simulink model "EX4zadanie2"  (R2023b)
settings: Solver=FixedStepDiscrete  StartTime=0.0  StopTime=0.0  RelTol=1e-3
libraries: CPOiS_SourcesSinks x10, CPOiS_Filters x6, CPOiS_DataManipulation_DataTypeConversion x6, CPOiS_DataManipulation_IntroduceNoise x2
settings Model: Creator=kkarkosz  LastModifiedBy=alyskawa

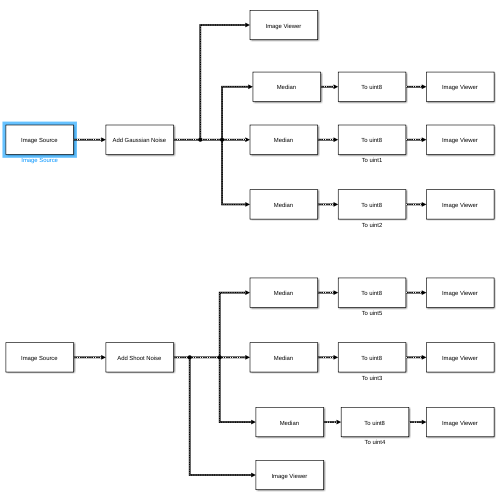
[thumbnail: Simulink's stored preview of the top-level diagram]
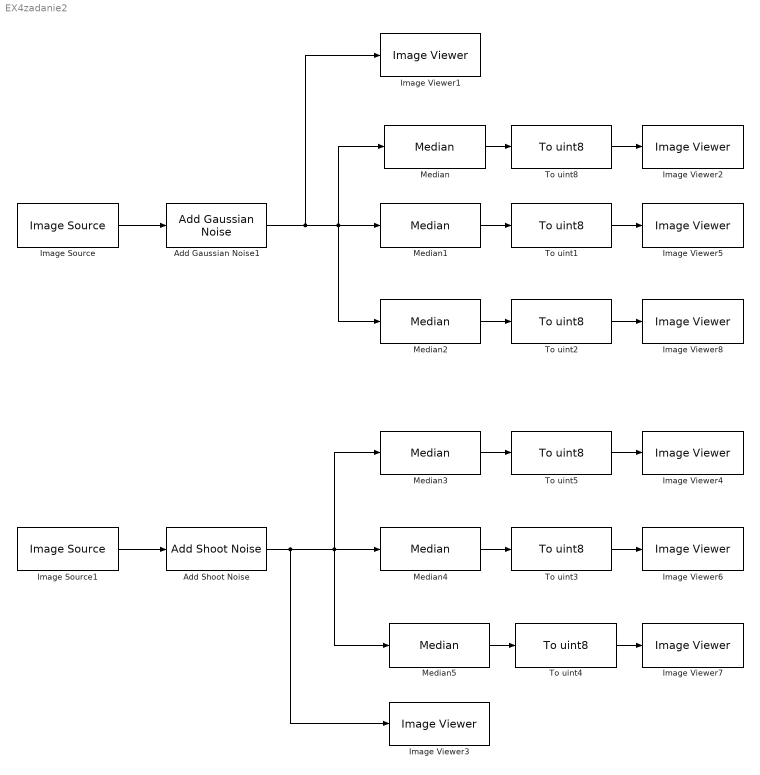
== system EX4zadanie2 ==
  Add Gaussian Noise1 : CPOiS_DataManipulation_IntroduceNoise/Add Gaussian Noise  Mean=10.0  Variance=1
      settings: SourceProductName=CPOiS - Digital image and signal processing
  Add Shoot Noise : CPOiS_DataManipulation_IntroduceNoise/Add Shoot Noise  Density=10
      settings: SourceProductName=CPOiS - Digital image and signal processing
  Image Source : CPOiS_SourcesSinks/Image Source  FileSelection=gull.png
      settings: SourceProductName=CPOiS - Digital image and signal processing
  Image Source1 : CPOiS_SourcesSinks/Image Source  FileSelection=gull.png
      settings: SourceProductName=CPOiS - Digital image and signal processing
  Image Viewer{1..8} (8 alike) : CPOiS_SourcesSinks/Image Viewer
      settings: SourceProductName=CPOiS - Digital image and signal processing
  Median{,1..5} (6 alike) : CPOiS_Filters/Median
      settings: SourceProductName=CPOiS - Digital image and signal processing
  To uint{1..5,8} (6 alike) : CPOiS_DataManipulation_DataTypeConversion/To uint8
      settings: SourceProductName=CPOiS - Digital image and signal processing
  wires:
  Image Source/1 -> Add Gaussian Noise1/1
  Add Gaussian Noise1/1 -> Image Viewer1/1, Median1/1, Median/1, Median2/1
  To uint8/1 -> Image Viewer2/1
  To uint1/1 -> Image Viewer5/1
  To uint2/1 -> Image Viewer8/1
  Median2/1 -> To uint2/1
  Median/1 -> To uint8/1
  Median1/1 -> To uint1/1
  Median5/1 -> To uint4/1
  To uint4/1 -> Image Viewer7/1
  Median4/1 -> To uint3/1
  Median3/1 -> To uint5/1
  To uint3/1 -> Image Viewer6/1
  To uint5/1 -> Image Viewer4/1
  Image Source1/1 -> Add Shoot Noise/1
  Add Shoot Noise/1 -> Image Viewer3/1, Median5/1, Median4/1, Median3/1
